simulink model "tests_control_franka"  (R2020b)
settings: Solver=ode1  StartTime=0.0  StopTime=5  FixedStep=0.001  RelTol=1e-4
values from neighbouring files (symbols this model uses):
  a0 = 0.99    [init.m]
  berta = 0.98    [init.m]
  csi = 1    [init.m]
  e_max = 0.01    [init.m]
  F_int_max = 5    [init.m]
  F_max = 2    [init.m]
  M = 1    [init.m]
  mass = 1    [init.m]
  q_max = q_max - deg2rad([0 0 0 10 0 5 0])    [init.m]
  q_min = q_min + deg2rad([0 0 0 10 0 5 0])    [init.m]
libraries: simulink x4
(part 2 of 2)

== matlab function tests_control_franka/PLANNER2/KX_GENERATOR ==
  settings: updateMethod=DISCRETE  sampleTime=Ts
  data: k output; F_ext input; z input; z_des input; dz_des input; int input; comp input; e_max parameter; F_max parameter; F_int_max parameter
function k = fcn(F_ext, z, z_des, dz_des, int, comp, e_max, F_max, F_int_max)
%% Description
% Set the K coefficient for a variable impedance controller based on a
% desired trajectory

%% Outputs
% k             stiffness

%% Inputs
% F_ext         measured external force
% z_des         desired trajectory
% z             current position
% int, comp     booleans for the interaction and compensation phase

%% Parameters
% F_int_max     desired interaction force
% F_max         nominal disturbance forces
% e_max         maximum steady-state error

%% persistent initialization
persistent ki kc F_comp int_prec comp_prec z_int z_int_dir set_F_comp
if isempty(ki)
   ki = F_max/e_max;        % k obtained from interaction
end
if isempty(F_comp)
   F_comp = 0;              % weight to compensate
end
if isempty(kc)
      kc = F_max/e_max;     % k obtained from compensation
end
if isempty(z_int) 
    z_int = 1000;       % obstacle(or interaction) position
end
if isempty(z_int_dir) 
    z_int_dir = 0;          % prohibited direction due to the obstacle
end
if isempty(int_prec)
    int_prec = 0;           % previous values of int
end
if isempty(comp_prec)
    comp_prec = 0;          % previous values od comp
end
if isempty(set_F_comp)
    set_F_comp = 1;
end
%% INTERACTION
% set ki in order to match a desired interaction force with the
% envirorment, and store interaction's position when detected
% X axes
if int == 1
    % detection of an interaction 
    if abs(F_ext-F_comp) > F_max
        if z_int == 1000                     % z_int has not been set yet
            z_int = z;
            z_int_dir = -sign(F_ext-F_comp);
            set_F_comp = 0; 
        end
    end
    % setting of ki
    if abs(F_ext-F_comp) > F_int_max 
        % if interaction force is higher than threshold
        if ki*abs(z-z_des) > F_int_max
            ktemp_x = F_int_max/abs(z-z_des);
            if ktemp_x < ki                % ki needs to be only decreased
                ki = ktemp_x;
            end
        end
    end
end

%% COMPENSATION
% set kc in order to compensate the effect of the weight of the object,
% and store it
% X axes
if comp == 1
    % compensation detection
    if z_int == 1000                     % z_int not set before
        if abs(F_ext)/kc > e_max         
            kc = abs(F_ext)/e_max;
            if set_F_comp > 0.1
                F_comp = F_ext;
            end
        end
    else 
        if z_int_dir == 1                % obstacle in above
            if z < z_int
                if abs(F_ext)/kc > e_max 
                    kc = abs(F_ext)/e_max;
                    if set_F_comp > 0.1
                        F_comp = F_ext;
                    end
                end
            end
        else                                % obstacle is below
            if z > z_int
                if abs(F_ext)/kc > e_max
                    kc = abs(F_ext)/e_max;
                    if set_F_comp > 0.1
                        F_comp = F_ext;
                    end
                end
            end
        end 
   end
end

%% reset to default values when comp or int shifts to zero
if comp==0 && comp_prec==1
    kc = F_max/e_max;
    F_comp = 0;
    set_F_comp = 0;
end
if int==0 && int_prec==1
    ki = F_max/e_max;
end

%% from int to comp and vice versa
if int==1 && int_prec==0
    if comp_prec == 1
        ki = kc;
    end
    z_int=1000;
    z_int_dir=0;
end
if comp == 1 && comp_prec==0
    if int_prec == 1
        kc = ki;
    end
    set_F_comp = 1;
end

% update to last booleans
int_prec = int;
comp_prec = comp;


%% Selection of Final Values of D-K
% default values
k = abs(F_max)/e_max;

% compensation
if comp == 1
    k = kc;
end

% both compensation and interaction are activated
% if "away" from obstacle set k = kc else ki
if int == 1
    k = ki;
    if comp == 1
        if z_int == 1000
            k = kc;                       % obstacle not reached
        else
            if z_int_dir == 1
                if z_des < z_int
                    if sign(dz_des*z_int_dir) < 0
                        k = kc;               % obstacle reached but "going away"
                    end
                end
            else
                if z_des > z_int
                    if sign(dz_des*z_int_dir) < 0
                        k = kc;               % obstacle reached but "going away"
                    end
                end
            end
        end
    else
        if z_int == 1000
            k = F_max/e_max;            % restore to default
        else
            if z_int_dir == 1
                if z_des < z_int
                    k = F_max/e_max;    % restore because "going away"
                end
            else
                if z_des > z_int
                    k = F_max/e_max;    % restore because "going away"
                end
            end
        end
    end
end

end

== matlab function tests_control_franka/PLANNER2/KZ_GENERATOR ==
  settings: updateMethod=DISCRETE  sampleTime=Ts
  data: k output; F_ext input; z input; z_des input; dz_des input; int input; comp input; e_max parameter; F_max parameter; F_int_max parameter
function k = fcn(F_ext, z, z_des, dz_des, int, comp, e_max, F_max, F_int_max)
%% Description
% Set the K coefficient for a variable impedance controller based on a
% desired trajectory

%% Outputs
% k             stiffness

%% Inputs
% F_ext         measured external force
% z_des         desired trajectory
% z             current position
% int, comp     booleans for the interaction and compensation phase

%% Parameters
% F_int_max     desired interaction force
% F_max         nominal disturbance forces
% e_max         maximum steady-state error

%% persistent initialization
persistent ki kc F_comp int_prec comp_prec z_int z_int_dir set_F_comp
if isempty(ki)
   ki = F_max/e_max;        % k obtained from interaction
end
if isempty(F_comp)
   F_comp = 0;              % weight to compensate
end
if isempty(kc)
      kc = F_max/e_max;     % k obtained from compensation
end
if isempty(z_int) 
    z_int = 1000;       % obstacle(or interaction) position
end
if isempty(z_int_dir) 
    z_int_dir = 0;          % prohibited direction due to the obstacle
end
if isempty(int_prec)
    int_prec = 0;           % previous values of int
end
if isempty(comp_prec)
    comp_prec = 0;          % previous values od comp
end
if isempty(set_F_comp)
    set_F_comp = 1;
end
%% INTERACTION
% set ki in order to match a desired interaction force with the
% envirorment, and store interaction's position when detected
% X axes
if int == 1
    % detection of an interaction 
    if abs(F_ext-F_comp) > F_max
        if z_int == 1000                     % z_int has not been set yet
            z_int = z;
            z_int_dir = -sign(F_ext-F_comp);
            set_F_comp = 0; 
        end
    end
    % setting of ki
    if abs(F_ext-F_comp) > F_int_max 
        % if interaction force is higher than threshold
        if ki*abs(z-z_des) > F_int_max
            ktemp_x = F_int_max/abs(z-z_des);
            if ktemp_x < ki                % ki needs to be only decreased
                ki = ktemp_x;
            end
        end
    end
end

%% COMPENSATION
% set kc in order to compensate the effect of the weight of the object,
% and store it
% X axes
if comp == 1
    % compensation detection
    if z_int == 1000                     % z_int not set before
        if abs(F_ext)/kc > e_max         
            kc = abs(F_ext)/e_max;
            if set_F_comp > 0.1
                F_comp = F_ext;
            end
        end
    else 
        if z_int_dir == 1                % obstacle in above
            if z < z_int
                if abs(F_ext)/kc > e_max 
                    kc = abs(F_ext)/e_max;
                    if set_F_comp > 0.1
                        F_comp = F_ext;
                    end
                end
            end
        else                                % obstacle is below
            if z > z_int
                if abs(F_ext)/kc > e_max
                    kc = abs(F_ext)/e_max;
                    if set_F_comp > 0.1
                        F_comp = F_ext;
                    end
                end
            end
        end 
   end
end

%% reset to default values when comp or int shifts to zero
if comp==0 && comp_prec==1
    kc = F_max/e_max;
    F_comp = 0;
    set_F_comp = 0;
end
if int==0 && int_prec==1
    ki = F_max/e_max;
end

%% from int to comp and vice versa
if int==1 && int_prec==0
    if comp_prec == 1
        ki = kc;
    end
    z_int=1000;
    z_int_dir=0;
end
if comp == 1 && comp_prec==0
    if int_prec == 1
        kc = ki;
    end
    set_F_comp = 1;
end

% update to last booleans
int_prec = int;
comp_prec = comp;


%% Selection of Final Values of D-K
% default values
k = abs(F_max)/e_max;

% compensation
if comp == 1
    k = kc;
end

% both compensation and interaction are activated
% if "away" from obstacle set k = kc else ki
if int == 1
    k = ki;
    if comp == 1
        if z_int == 1000
            k = kc;                       % obstacle not reached
        else
            if z_int_dir == 1
                if z_des < z_int
                    if sign(dz_des*z_int_dir) < 0
                        k = kc;               % obstacle reached but "going away"
                    end
                end
            else
                if z_des > z_int
                    if sign(dz_des*z_int_dir) < 0
                        k = kc;               % obstacle reached but "going away"
                    end
                end
            end
        end
    else
        if z_int == 1000
            k = F_max/e_max;            % restore to default
        else
            if z_int_dir == 1
                if z_des < z_int
                    k = F_max/e_max;    % restore because "going away"
                end
            else
                if z_des > z_int
                    k = F_max/e_max;    % restore because "going away"
                end
            end
        end
    end
end

end

== matlab function tests_control_franka/direct kinematics2 ==
  data: q_dot input double; q input double; z output double; dz output double; or output
function [z,dz,or] = fcn(q_dot,q)
coder.extrinsic('get_Ja');
% persistent dh_c
% if isempty(dh_c)
%     dh_c = Load_Franka_DH();
% end
[DH, Conv] = Load_Franka_DH();
z = zeros(3,1);
%z = get_pos(q);

[p,R] = DirectKinematic(DH,[q;0],Conv);
z = p;
phi = atan2(R(2,1),R(1,1));
teta = atan2(-R(3,1),sqrt(R(3,2)^2 + R(3,3)^2)); 
psi = atan2(R(3,2),R(3,3));
or = [phi teta psi]';

Ja = zeros(6,7);
Ja = get_Ja(q);

dz = zeros(3,1);
dz = Ja(1:3,1:7)*q_dot;

end

== matlab function tests_control_franka/null_space_controller1 ==
  settings: updateMethod=DISCRETE  sampleTime=Ts
  data: time input; q input; tau output; q_dot input
function tau = nsc(time,q, q_dot)
coder.extrinsic('get_Ja','get_MassMatrix');
Ja = zeros(6,7);
B = zeros(7,7);
q_min = [-2.8973   -1.7628   -2.8973   -3.0718   -2.8973   -0.0175  -2.8973];
q_min = q_min + deg2rad([0 0 0 10 0 5 0]);
%        166.0031  101.0010  166.0031 -3.9992   166.0031   215.0024  166.0031
q_max = [ 2.8973    1.7628    2.8973  -0.0698    2.8973    3.7525    2.8973];
q_max = q_max - deg2rad([0 0 0 10 0 5 0]);

q_des = (q_max + q_min)'/2;

Ja = get_Ja(q);
Ja(isnan(Ja)) = 0;
B = get_MassMatrix(q);
B_inv = inv(B);
%Ja_inv = inv(B)*(Ja')*inv(Ja*inv(B)*Ja');
Ja_t_inv = inv(Ja*B_inv*Ja')*Ja*B_inv; %inertia-weighted pseudo inverse Ja'
Ja_t_inv(isnan(Ja_t_inv)) = 0;
%Ja_t_inv = inv(Ja*Ja')*Ja;
%Ja_inv = Ja_t_inv'; 
% add joint friction
D_joints = eye(7)*2;
K_joints = eye(7)*10;
%N = eye(7) - Ja_inv*Ja;
N = eye(7) - Ja'*(Ja_t_inv);
tau = N*(K_joints*(q_des - q) -D_joints*q_dot);
end

== matlab function tests_control_franka/TRAJECTORY2/GENERATOR ==
  data: time input; z_des output; dz_des output; ddz_des output; or_des output; int output; comp output
function  [z_des, dz_des, ddz_des, or_des, int, comp] = fcn(time)
coder.extrinsic('wrapToPi')
t= time;
int = [0; 0; 0];
comp = [0; 0; 0];
q = [0; pi/4; 0; -pi/2; 0; 0; 0];
or_init = zeros(3,1);
or_init = wrapToPi([-3.14;0.78+pi/4;0]);
pos_init = [0.35; 0; 0.3];
or_des = or_init;
%or_des = or_init + [0;0;t];
or_des = wrapToPi(or_des);

z_des = pos_init + [0; sin(2*t)/4; sin(4*t)/8];
dz_des = [0; cos(2*t)/2; +cos(4*t)/4];
ddz_des = [0; -sin(2*t); -sin(4*t)*2];

end

== matlab function tests_control_franka/TRAJECTORY3/GENERATOR ==
  data: time input; z_des output; dz_des output; ddz_des output; or_des output; int output; comp output
function  [z_des, dz_des, ddz_des, or_des, int, comp] = fcn(time)
coder.extrinsic('wrapToPi')
t= time;
int = [0; 0; 0];
comp = [0; 0; 0];
q = [0; pi/4; 0; -pi/2; 0; 0; 0];
or_init = zeros(3,1);
or_init = wrapToPi([-3.14;0.78+pi/4;0]);
pos_init = [0.35; 0; 0.3];
or_des = or_init;
or_des = wrapToPi(or_des);

z_des = pos_init + [sin(2*t)/4; sin(4*t)/8; 0];
dz_des = [cos(2*t)/2; +cos(4*t)/4; 0];
ddz_des = [-sin(2*t); -sin(4*t)*2; 0];

end

== matlab function tests_control_franka/TRAJECTORY4/GENERATOR ==
  data: time input; z_des output; dz_des output; ddz_des output; or_des output; int output; comp output
function  [z_des, dz_des, ddz_des, or_des, int, comp] = fcn(time)
coder.extrinsic('wrapToPi')
t= time;
int = [0; 0; 0];
comp = [0; 0; 0];
% da copiare q nel blocco initial condition di simulink
q = [0; pi/4; 0; -pi/2; 0; deg2rad(135); 0];
or_init = zeros(3,1);
or_init = wrapToPi([0;0;pi]);     % Rotazioni Z, Y, X
pos_init = [0.47; 0; 0.29];
or_des = or_init;
or_des = wrapToPi(or_des);

z_des = pos_init + [sin(4*t)/8; sin(2*t)/4; t/20];
dz_des = [cos(4*t)/2; +cos(2*t)/2; 1/20];
ddz_des = [-sin(4*t)*2; -sin(2*t); 0];

end

== matlab function tests_control_franka/TRAJECTORY5/GENERATOR ==
  data: time input; z_des output; dz_des output; ddz_des output; or_des output; int output; comp output
function  [z_des, dz_des, ddz_des, or_des, int, comp] = fcn(time)
coder.extrinsic('wrapToPi')
t= time;
int = [0; 0; 0];
comp = [0; 0; 0];
% da copiare q nel blocco initial condition di simulink
q = [0; pi/4; 0; -pi/2; 0; deg2rad(135); 0];
or_init = zeros(3,1);
or_init = wrapToPi([0;0;pi]);     % Rotazioni Z, Y, X
pos_init = [0.47; 0; 0.29];
or_des = or_init;
or_des = wrapToPi(or_des);

z_des = pos_init + [sin(4*t)/8; sin(2*t)/4; sin(20*t)/20];
dz_des = [cos(4*t)/2; +cos(2*t)/2; cos(20*t)];
ddz_des = [-sin(4*t)*2; -sin(2*t); -sin(20*t)*20];

end

== matlab function tests_control_franka/PLANNER1/KD_INTERPOLATOR  ==
  settings: updateMethod=DISCRETE  sampleTime=Ts
  data: time input; K output; kx_f input; ky_f input; kz_f input; D output; e_max parameter; F_max parameter; M parameter; berta parameter; a0 parameter; mass parameter; csi parameter
function [K,D] = fcn(time, kx_f, ky_f, kz_f, e_max, F_max, M, berta, a0, mass, csi)
%% Description
% Interpolate K in order to guarantee stability

%% Outputs
% K             Stiffness matrix
% D             Damping matrix

%% Inputs
% kx_f, ky, f   desired values of K

%% Parameters
% F_max         nominal disturbance forces
% e_max         maximum steady-state error
% M             virtual mass
% berta, a0     parameters for the computation of stability conditions
% mass          virtual mass

%% persistent initialization
persistent kx ky kz time_prec
if isempty(time_prec)
    time_prec = 0;              % previous simulation time
end
if isempty(kx)
   kx = F_max/e_max;         % last value of k
end
if isempty(ky)
   ky = F_max/e_max;
end
if isempty(kz)
   kz = F_max/e_max;
end

% set k from desired one 
if kx_f <= kx       
    kx = kx_f;
else 
    % increese k in accordance with the stability conditions
    kx_i = kx;
    k_dotx = berta*(4*a0*sqrt(kx_i/mass)*(kx_i)^(3/2))/(sqrt(kx_i) + 2*a0*csi*sqrt(kx_i));
    k_tempx = kx_i + k_dotx*(time -time_prec);
    if k_tempx > kx_f
        kx = kx_f;
    else
        kx = k_tempx;
    end
end

% Y axes, same as X axes
if ky_f <= ky
    ky = ky_f;
else 
    ky_i = ky;
    k_doty = berta*(4*a0*sqrt(ky_i/mass)*(ky_i)^(3/2))/(sqrt(ky_i) + 2*a0*csi*sqrt(ky_i));
    k_tempy = ky_i + k_doty*(time -time_prec);
    if k_tempy > ky_f
        ky = ky_f;
    else
        ky = k_tempy;
    end
end

% Z axes, same as other axes
if kz_f <= kz
    kz = kz_f;
else 
    kz_i = kz;
    k_dotz = berta*(4*a0*sqrt(kz_i/mass)*(kz_i)^(3/2))/(sqrt(kz_i) + 2*a0*csi*sqrt(kz_i));
    k_tempz = kz_i + k_dotz*(time -time_prec);
    if k_tempz > kz_f
        kz = kz_f;
    else
        kz = k_tempz;
    end
end

time_prec = time;

% damping computation, critically damped condition
dx = sqrt(4*kx*M);
dy = sqrt(4*ky*M);
dz = sqrt(4*kz*M);

%% Final impedance matrices
D = diag([dx, dy, dz]);
K = diag([kx, ky, kz]);

end
